simulink model "Modulador_trifasico_de_tension"  (R2023b)
settings: Solver=VariableStepAuto  StartTime=0.0  StopTime=10.0  RelTol=1e-3
undefined symbols (not defined in the file): magnitude, Vsat, w_n_modulador, zeta_mod
settings Model: Creator=tomas  LastModifiedBy=tomas

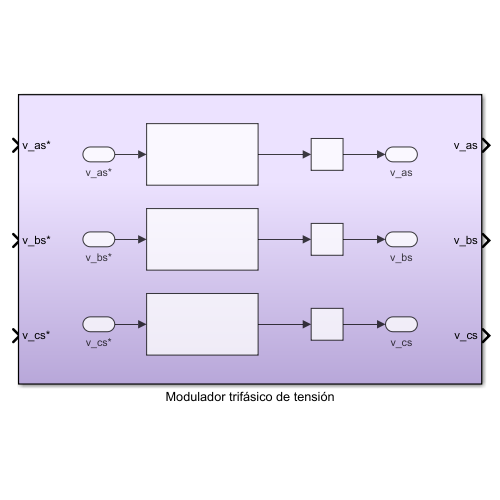
[thumbnail: Simulink's stored preview of the top-level diagram]
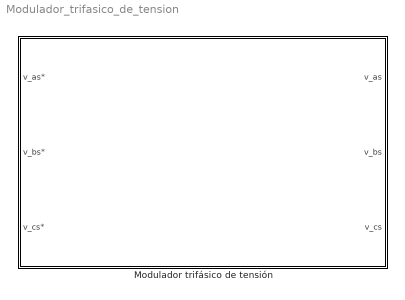
== system Modulador_trifasico_de_tension ==
  Modulador trifásico de tensión : Subsystem

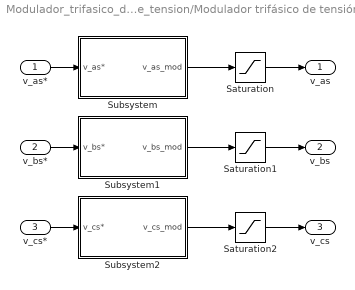
== system Modulador_trifasico_de_tension/Modulador trifásico de tensión ==
  v_as* : Inport
  v_bs* : Inport  Port=2
  v_cs* : Inport  Port=3
  Saturation : Saturate  UpperLimit=Vsat  LowerLimit=-Vsat
  Saturation1 : Saturate  UpperLimit=Vsat  LowerLimit=-Vsat
  Saturation2 : Saturate  UpperLimit=Vsat  LowerLimit=-Vsat
  Subsystem : Subsystem
  Subsystem1 : Subsystem
  Subsystem2 : Subsystem
  v_as : Outport
  v_bs : Outport  Port=2
  v_cs : Outport  Port=3
  wires:
  Subsystem/1(v_as_mod) -> Saturation/1
  Subsystem1/1(v_bs_mod) -> Saturation1/1
  Subsystem2/1(v_cs_mod) -> Saturation2/1
  v_cs*/1 -> Subsystem2/1(v_cs*)
  v_bs*/1 -> Subsystem1/1(v_bs*)
  v_as*/1 -> Subsystem/1(v_as*)
  Saturation/1 -> v_as/1
  Saturation1/1 -> v_bs/1
  Saturation2/1 -> v_cs/1

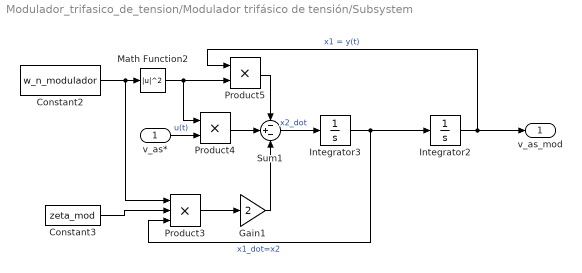
== system Modulador_trifasico_de_tension/Modulador trifásico de tensión/Subsystem ==
  v_as* : Inport
  Constant2 : Constant  Value=w_n_modulador
  Constant3 : Constant  Value=zeta_mod
  Gain1 : Gain  Gain=2
  Integrator2 : Integrator
  Integrator3 : Integrator
  Math Function2 : Math  Operator=magnitude^2
  Product3 : Product  Inputs=3
  Product4 : Product
  Product5 : Product
  Sum1 : Sum  Inputs=-+-
  v_as_mod : Outport
  wires:
  Math Function2/1 -> Product5/2, Product4/1
  Integrator3/1 -> Product3/3, Integrator2/1  "x1_dot=x2"
  v_as*/1 -> Product4/2  "u(t)"
  Product4/1 -> Sum1/2
  Sum1/1 -> Integrator3/1  "x2_dot"
  Integrator2/1 -> v_as_mod/1, Product5/1  "x1 = y(t)"
  Gain1/1 -> Sum1/3
  Product3/1 -> Gain1/1
  Constant2/1 -> Product3/1, Math Function2/1
  Product5/1 -> Sum1/1
  Constant3/1 -> Product3/2

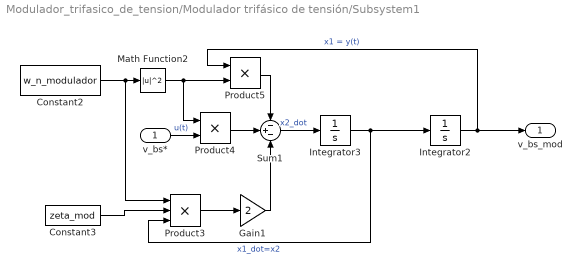
== system Modulador_trifasico_de_tension/Modulador trifásico de tensión/Subsystem1 ==
  v_bs* : Inport
  Constant2 : Constant  Value=w_n_modulador
  Constant3 : Constant  Value=zeta_mod
  Gain1 : Gain  Gain=2
  Integrator2 : Integrator
  Integrator3 : Integrator
  Math Function2 : Math  Operator=magnitude^2
  Product3 : Product  Inputs=3
  Product4 : Product
  Product5 : Product
  Sum1 : Sum  Inputs=-+-
  v_bs_mod : Outport
  wires:
  Math Function2/1 -> Product5/2, Product4/1
  Integrator3/1 -> Product3/3, Integrator2/1  "x1_dot=x2"
  v_bs*/1 -> Product4/2  "u(t)"
  Product4/1 -> Sum1/2
  Sum1/1 -> Integrator3/1  "x2_dot"
  Integrator2/1 -> v_bs_mod/1, Product5/1  "x1 = y(t)"
  Gain1/1 -> Sum1/3
  Product3/1 -> Gain1/1
  Constant2/1 -> Product3/1, Math Function2/1
  Product5/1 -> Sum1/1
  Constant3/1 -> Product3/2

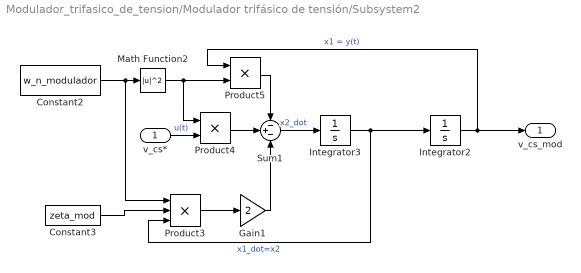
== system Modulador_trifasico_de_tension/Modulador trifásico de tensión/Subsystem2 ==
  v_cs* : Inport
  Constant2 : Constant  Value=w_n_modulador
  Constant3 : Constant  Value=zeta_mod
  Gain1 : Gain  Gain=2
  Integrator2 : Integrator
  Integrator3 : Integrator
  Math Function2 : Math  Operator=magnitude^2
  Product3 : Product  Inputs=3
  Product4 : Product
  Product5 : Product
  Sum1 : Sum  Inputs=-+-
  v_cs_mod : Outport
  wires:
  Math Function2/1 -> Product5/2, Product4/1
  Integrator3/1 -> Product3/3, Integrator2/1  "x1_dot=x2"
  v_cs*/1 -> Product4/2  "u(t)"
  Product4/1 -> Sum1/2
  Sum1/1 -> Integrator3/1  "x2_dot"
  Integrator2/1 -> v_cs_mod/1, Product5/1  "x1 = y(t)"
  Gain1/1 -> Sum1/3
  Product3/1 -> Gain1/1
  Constant2/1 -> Product3/1, Math Function2/1
  Product5/1 -> Sum1/1
  Constant3/1 -> Product3/2
